simulink model "DC_Motor"  (R2021b)
settings: Solver=VariableStepAuto  StartTime=0.0  StopTime=10.0  RelTol=1e-3
model workspace (MAT data in the model file):
  B = 0.02
  J = 7
  K = 1.4
  L = 0.1
  R = 0.4
  TL = 5
  Vin = 12
undefined symbols (not defined in the file): sigbuilder_block
settings Model: Creator=amr_y  LastModifiedBy=amr_y

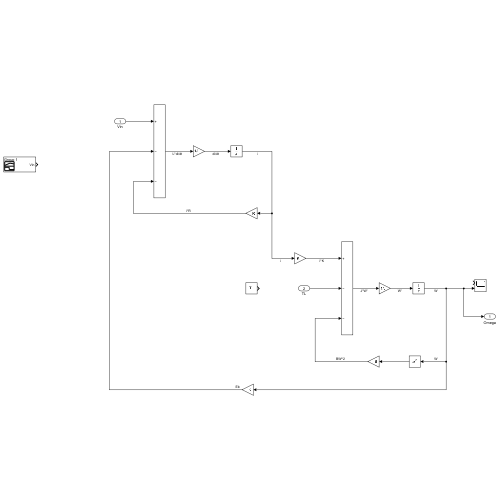
[thumbnail: Simulink's stored preview of the top-level diagram]
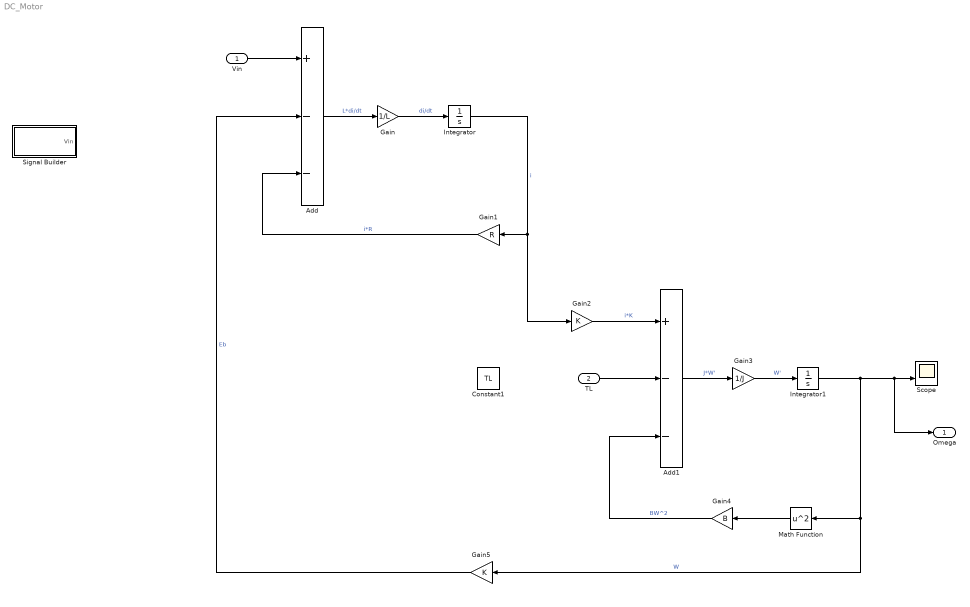
== system DC_Motor ==
  Vin : Inport
  TL : Inport  Port=2
  Add : Sum  Inputs=+--
  Add1 : Sum  Inputs=+--
  Constant1 : Constant  Value=TL
  Gain : Gain  Gain=1/L
  Gain1 : Gain  Gain=R
  Gain2 : Gain  Gain=K
  Gain3 : Gain  Gain=1/J
  Gain4 : Gain  Gain=B
  Gain5 : Gain  Gain=K
  Integrator : Integrator
  Integrator1 : Integrator
  Math Function : Math  Operator=square  SaturateOnIntegerOverflow=on
  Scope : Scope  NumInputPorts=2
  Signal Builder : Subsystem  Tag=STV Subsys  LoadFcn=sigbuilder_block('load');  StartFcn=sigbuilder_block('start');  StopFcn=sigbuilder_block('stop');  ClipboardFcn=sigbuilder_block('clipboard');  mask(Sigbuilder block){tuvar=[0:10]}
      mask help: Simulink:masks:SigbuilderBlock_MD
      mask init:
      | if ~strcmp(get_param(bdroot(gcbh),'SimulationStatus'),'stopped') tuvar = sigbuilder_block('maskInit'); end
      settings: CopyFcn=sigbuilder_block('copy');  DeleteFcn=sigbuilder_block('delete');  ModelCloseFcn=sigbuilder_block('modelClose');  PreSaveFcn=sigbuilder_block('preSave');  PauseFcn=sigbuilder_block('pause');  ContinueFcn=sigbuilder_block('continue');  NameChangeFcn=sigbuilder_block('namechange');  OpenFcn=sigbuilder_block('open',[437.6 199.2 550.4 400 ]);  CloseFcn=sigbuilder_block('close');
      mask Display: plot(0, 0, 100, 100,[2, 2, 32, 32, 2], [68, 8, 8, 68, 68],[32, 2], [38, 38], [32, 19, 2],[53, 60, 44], [32, 17, 17, 2],[16, 16, 31, 31]);txt = getActiveGroup(gcbh);text(2, 100, txt,'verticalAlignment', 'top');
  Omega : Outport
  wires:
  Add/1 -> Gain/1  "L*di/dt"
  Gain/1 -> Integrator/1  "di/dt"
  Integrator/1 -> Gain1/1, Gain2/1  "i"
  Gain1/1 -> Add/3  "i*R"
  Gain2/1 -> Add1/1  "i*K"
  Add1/1 -> Gain3/1  "J*W'"
  Gain3/1 -> Integrator1/1  "W'"
  Integrator1/1 -> Gain5/1, Math Function/1, Omega/1, Scope/2  "W"
  Math Function/1 -> Gain4/1
  Gain4/1 -> Add1/3  "BW^2"
  Gain5/1 -> Add/2  "Eb"
  Vin/1 -> Add/1
  TL/1 -> Add1/2

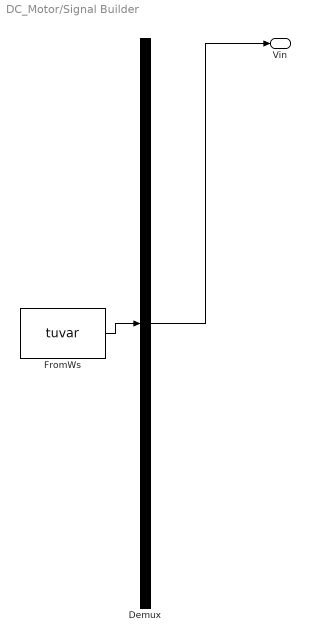
== system DC_Motor/Signal Builder ==
  Demux : Demux  Tag=STV Demux  Outputs=1
      settings: DisplayOption=none
  FromWs : FromWorkspace  Tag=STV FromWs  VariableName=tuvar
      SigBuilderData=|
      | common.afterFinalStr = 'Extrapolate'
      | common.sampleTime = 0
      | dataSet.timeRange = [0 10]
      | dataSet.name = 'Group 1'
      | sbobj.Groups.Name = 'Group 1'
      | sbobj.Groups.Signals.Name = 'Vin'
      | sbobj.Groups.Signals.XData = [0 2 2 4 4 6 6 8 8 10]
      | sbobj.Groups.Signals.YData = [5 5 15 15 25 25 10 10 30 30]
  Vin : Outport  Tag=STV Outport
  wires:
  Demux/1 -> Vin/1
  FromWs/1 -> Demux/1
